simulink model "cell_sim"  (R2022a)
settings: Solver=VariableStepAuto  StartTime=0.0  StopTime=10000  RelTol=1e-3
undefined symbols (not defined in the file): T_AMB
libraries: ee_lib x2, fl_lib x2, simulink x2, nesl_utility x1
settings Model: DataDictionary=battery.sldd  Creator=Cristobal  LastModifiedBy=Cristobal
settings SFSimCC: SimTargetLang=C++  GPUAcceleration=on  SimDLTargetLibrary=cudnn

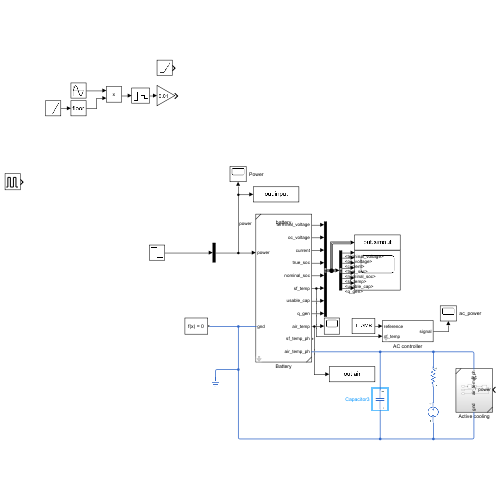
[thumbnail: Simulink's stored preview of the top-level diagram]
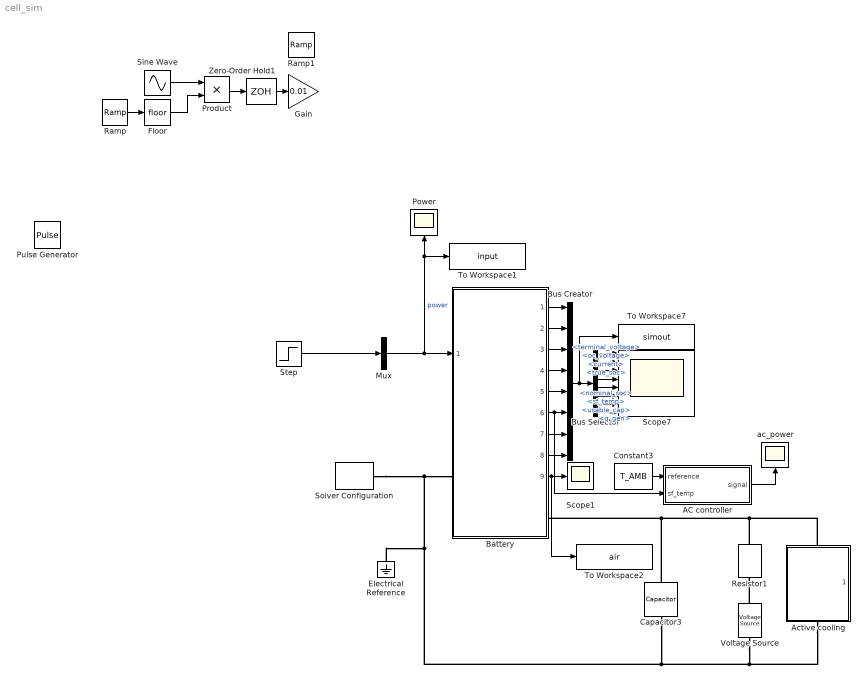
== system cell_sim ==
  AC controller : Subsystem  mask{KP=100, KI=10}
      mask prompts: KP "P"; KI "K"
      mask DialogControl ParameterGroupVar Prompt: Gains
  Active cooling : Subsystem  ReferencedSubsystem=ac
      settings: PortSchema="{\"entries\":[{\"content\":{\"sides\":[{\"content\":{\"connectorIds\":[]},\"type\":\"ConnectorPlacement.EquallySpacedRectSide\",\"uuid\":\"5ed7fd81-1699-43d1-ba74-6b7eb013c598\"},{\"content\":{\"connectorIds\":[\"In1\"],\"side\":\"RIGHT\"},\"type\":\"ConnectorPlacement.EquallySpacedRectSide\",\"uuid\":\"4fe335e4-955c-4431-8200-89d4c6c9e1a1\"},{\"content\":{\"connectorIds\":[\"LConn1\"],\"side\":\"TOP\"},\"type\":\"ConnectorPlacement.EquallySpacedRectSide\",\"uuid\":\"87d46851-78c3-4bfa-a568-c2525415f646\"},{\"content\":{\"connectorIds\":[\"LConn2\"],\"side\":\"BOTTOM\"},\"type\":\"ConnectorPlacement.EquallySpacedRectSide\",\"uuid\":\"8344fc10-9b43-454f-b29e-8ffb41f614cd\"}]},\"type\":\"ConnectorPlacement.EquallySpacedConnector\",\"uuid\":\"bceebb64-3e01-4f52-89f3-41a2b35b670e\"}],\"packageUris\":[\"http://schema.mathworks.com/mf0/Connector/R2020b\"],\"version\":\"1.0\"}"
  Battery : Subsystem  ReferencedSubsystem=battery  initial_sf_temp=298  initial_soc=1  initial_soh=1
  Bus Creator : BusCreator  Inputs=8
  Bus Selector : BusSelector  OutputSignals=terminal_voltage,oc_voltage,current,true_soc,nominal_soc,sf_temp,usable_cap,q_gen
  Capacitor3 : ee_lib/Passive/Capacitor  cap_option=0  c=100 F  Cvec=[1e-05, 1e-06] F  Vvec=[0, 10] V  CV_table_symmetry=1  f_vec=[1, 10] kHz  DFext_vec=[.8, 1.2]  enable_C_tol=0  C_tol=5  tol_distribution=1  nSigma=4  r=0 Ohm  g=0 1/Ohm  averaging_period=0 s  enable_operating_limits=0  operating_limit_action=2  max_working_voltage_range=[-25, 25] V  power_rating=1 W  enable_faults=0  fault_action=1  Cscale_faulted=100  R_faulted=1e-3 Ohm  G_faulted=0 1/Ohm  tau_fault=1e-3 s  enable_temporal_fault=0  t_fault=1 s  enable_behavioral_fault=0  max_permissible_voltage_range=[-100, 100] V  t_fail_on_voltage=1 s  i_specify=off  i_priority=None  i=0 A  i_nominal_specify=off  i_nominal_unit=A  i_nominal_value=1  v_specify=off  v_priority=None  v=303 V  v_nominal_specify=off  v_nominal_unit=V  v_nominal_value=1  vc_specify=on  vc_priority=High  vc=T_AMB V  vc_nominal_specify=off  vc_nominal_unit=V  vc_nominal_value=1
  Constant3 : Constant  Value=T_AMB
  Electrical Reference : fl_lib/Electrical/Electrical Elements/Electrical Reference
      settings: SourceProductBaseCode=PW,SS,VE
  Floor : Rounding
  Gain : Gain  Gain=0.01
  Mux : Mux  Inputs=1
  Power : Scope
  Product : Product
  Pulse Generator : DiscretePulseGenerator  PulseType=Time based  Amplitude=60  Period=300  PulseWidth=50
  Ramp : simulink/Sources/Ramp  slope=1 / 60  start=0  InitialOutput=0
  Ramp1 : simulink/Sources/Ramp  slope=1 / 60000  start=0  InitialOutput=0
  Resistor1 : fl_lib/Electrical/Electrical Elements/Resistor  R=10 Ohm  i_specify=off  i_priority=None  i=0 A  i_nominal_specify=off  i_nominal_unit=A  i_nominal_value=1  v_specify=off  v_priority=None  v=0 V  v_nominal_specify=off  v_nominal_unit=V  v_nominal_value=1
      settings: SourceProductBaseCode=PW,SS,VE
  Scope1 : Scope
  Scope7 : Scope  NumInputPorts=8
  Sine Wave : Sin  Frequency=2 * pi / 60  Phase=pi / 2  SampleTime=0
  Solver Configuration : nesl_utility/Solver Configuration  PhysicalDomain=network_engine_domain  SubClassName=solver  LeftPortType=input  RightPortType=generic  Tones=[]  Harmonics=[]  SimulateNoise=off  Profile=off  UseLocalSampling=off  EnableSwitchedLinearOptims=on  FrequencyDomain=off  UseCCode=off  RelTol=0.001  AbsTol=0.001  MinStep=1e-09  ToWorkspace=off  RevertToSquareIcSolve=off  NumHomotopyIterations=100  PhasorMode=off  PhasorModeNumHarmonics=1  IndexReductionMethod=DerivativeReplacement  DoDC=off  ResidualTolerance=1e-09  UseLocalSolver=off  LocalSolverChoice=NE_BACKWARD_EULER_ADVANCER  LocalSolverSampleTime=0.001  DoFixedCost=off  MaxNonlinIter=3  MaxModeIter=2  ComputeImpulses=off  ImpulseIterations=2  LinearAlgebra=auto  LinearAlgebraNumThread=0  EquationFormulation=NE_TIME_EF  DelaysMemoryBudget=1024  AutomaticFiltering=on  FilteringTimeConstant=0.001  PartitionStorageMethod=AS_NEEDED  PartitionMemoryBudget=1024  PartitionMethod=ROBUST
      settings: SourceProductBaseCode=SS,PW,VE
  Step : Step  Time=500  Before=50  After=0  SampleTime=0
  To Workspace1 : ToWorkspace  VariableName=input  SaveFormat=Timeseries  SampleTime=-1
  To Workspace2 : ToWorkspace  VariableName=air  SaveFormat=Timeseries  SampleTime=-1
  To Workspace7 : ToWorkspace  VariableName=simout  SaveFormat=Timeseries  SampleTime=-1
  Voltage Source : ee_lib/Sources/Voltage Source  dc_voltage=T_AMB V  ac_voltage=0 V  ac_shift=0 rad  ac_frequency=60 Hz  noise_mode=0  PSD=0 V^2/Hz  repeatability=1  auto_seed=3499211588  user_seed=0  sample_time=1e-3 s  i_specify=off  i_priority=None  i=0 A  i_nominal_specify=off  i_nominal_unit=A  i_nominal_value=1  v_specify=off  v_priority=None  v=0 V  v_nominal_specify=off  v_nominal_unit=V  v_nominal_value=1
  Zero-Order Hold1 : ZeroOrderHold  SampleTime=30
  ac_power : Scope
  wires:
  Bus Creator/1 -> Bus Selector/1, To Workspace7/1
  Battery/3 -> Bus Creator/3
  Battery/4 -> Bus Creator/4
  Battery/5 -> Bus Creator/5
  Battery/6 -> AC controller/2(sf_temp), Bus Creator/6
  Battery/7 -> Bus Creator/7
  Battery/1 -> Bus Creator/1
  Battery/2 -> Bus Creator/2
  Bus Selector/1 -> Scope7/1  "<terminal_voltage>"
  Bus Selector/2 -> Scope7/2  "<oc_voltage>"
  Bus Selector/3 -> Scope7/3  "<current>"
  Bus Selector/4 -> Scope7/4  "<true_soc>"
  Bus Selector/5 -> Scope7/5  "<nominal_soc>"
  Bus Selector/6 -> Scope7/6  "<sf_temp>"
  Bus Selector/7 -> Scope7/7  "<usable_cap>"
  Battery/8 -> Bus Creator/8
  Mux/1 -> To Workspace1/1, Power/1, Battery/1  "power"
  Bus Selector/8 -> Scope7/8  "<q_gen>"
  Constant3/1 -> AC controller/1(reference)
  Sine Wave/1 -> Product/1
  Product/1 -> Zero-Order Hold1/1
  Ramp/1 -> Floor/1
  Floor/1 -> Product/2
  Zero-Order Hold1/1 -> Gain/1
  Battery/9 -> To Workspace2/1, Scope1/1
  AC controller/1(signal) -> ac_power/1
  Step/1 -> Mux/1
  connections:
  Electrical Reference/LConn1 -- Voltage Source/RConn1 -- Active cooling/LConn2 -- Capacitor3/RConn1 -- Solver Configuration/RConn1 -- Battery/LConn1
  Active cooling/LConn1 -- Capacitor3/LConn1 -- Battery/RConn2 -- Resistor1/LConn1
  Voltage Source/LConn1 -- Resistor1/RConn1

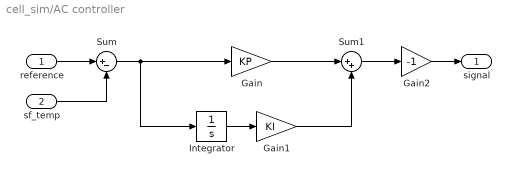
== system cell_sim/AC controller ==
  reference : Inport
  sf_temp : Inport  Port=2
  Gain : Gain  Gain=KP
  Gain1 : Gain  Gain=KI
  Gain2 : Gain  Gain=-1
  Integrator : Integrator
  Sum : Sum  Inputs=|+-  mask{KP=0}
  Sum1 : Sum  Inputs=|++
  signal : Outport
  wires:
  reference/1 -> Sum/1
  sf_temp/1 -> Sum/2
  Sum/1 -> Integrator/1, Gain/1
  Integrator/1 -> Gain1/1
  Gain/1 -> Sum1/1
  Gain1/1 -> Sum1/2
  Sum1/1 -> Gain2/1
  Gain2/1 -> signal/1
